simulink subsystem "ADCurve"  (R2023b)
settings: Solver=VariableStepAuto  StartTime=0.0  StopTime=10.0  RelTol=1e-3
settings Model: Creator=dfurodet  LastModifiedBy=dfurodet

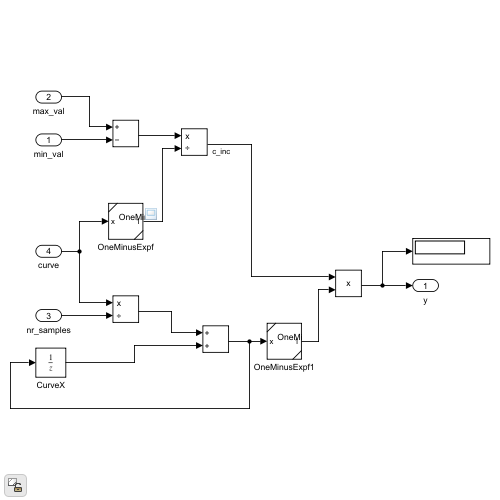
[thumbnail: Simulink's stored preview of the top-level diagram]
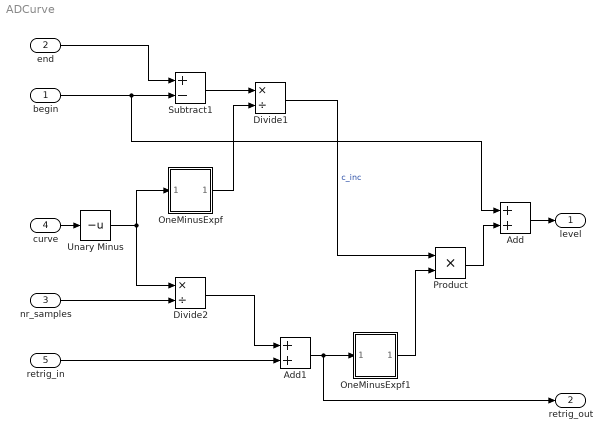
== system ADCurve ==
  begin : Inport
  end : Inport  Port=2
  nr_samples : Inport  Port=3
  curve : Inport  Port=4
  retrig_in : Inport  Port=5
  Add : Sum
  Add1 : Sum
  Divide1 : Product  Inputs=*/
  Divide2 : Product  Inputs=*/
  OneMinusExpf : Subsystem  ReferencedSubsystem=OneMinusExpf
  OneMinusExpf1 : Subsystem  ReferencedSubsystem=OneMinusExpf
  Product : Product
  Subtract1 : Sum  Inputs=+-
  Unary Minus : UnaryMinus
  level : Outport
  retrig_out : Outport  Port=2
  wires:
  end/1 -> Subtract1/1
  Subtract1/1 -> Divide1/1
  curve/1 -> Unary Minus/1
  Divide1/1 -> Product/1  "c_inc"
  Divide2/1 -> Add1/1
  nr_samples/1 -> Divide2/2
  Add1/1 -> retrig_out/1, OneMinusExpf1/1
  OneMinusExpf/1 -> Divide1/2
  OneMinusExpf1/1 -> Product/2
  begin/1 -> Subtract1/2, Add/1
  retrig_in/1 -> Add1/2
  Product/1 -> Add/2
  Add/1 -> level/1
  Unary Minus/1 -> Divide2/1, OneMinusExpf/1
